simulink model "lab4_E1"  (R2020a)
settings: Solver=FixedStepAuto  StartTime=0.0  StopTime=100  FixedStep=0.001  RelTol=1e-3
values from neighbouring files (symbols this model uses):
  y_r = 1    [lab8.mat]
undefined symbols (not defined in the file or in its folder): h, K, M, x_1_0, x_2_0, x_3_0
settings Model: Creator=bruno  LastModifiedBy=bruno

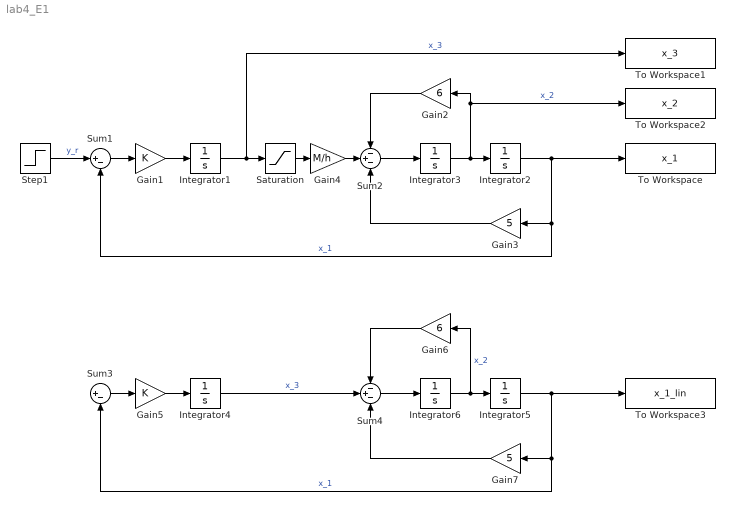
== system lab4_E1 ==
  Gain1 : Gain  Gain=K
  Gain2 : Gain  Gain=6
  Gain3 : Gain  Gain=5
  Gain4 : Gain  Gain=M/h
  Gain5 : Gain  Gain=K
  Gain6 : Gain  Gain=6
  Gain7 : Gain  Gain=5
  Integrator1 : Integrator  InitialCondition=x_3_0
  Integrator2 : Integrator  InitialCondition=x_1_0
  Integrator3 : Integrator  InitialCondition=x_2_0
  Integrator4 : Integrator  InitialCondition=x_3_0
  Integrator5 : Integrator  InitialCondition=x_1_0
  Integrator6 : Integrator  InitialCondition=x_2_0
  Saturation : Saturate  UpperLimit=h  LowerLimit=-h
  Step1 : Step  Time=0  After=y_r  SampleTime=0
  Sum1 : Sum  Inputs=|+-
  Sum2 : Sum  Inputs=-+-
  Sum3 : Sum  Inputs=|+-
  Sum4 : Sum  Inputs=-+-
  To Workspace : ToWorkspace  VariableName=x_1  SaveFormat=Timeseries  SampleTime=-1
  To Workspace1 : ToWorkspace  VariableName=x_3  SaveFormat=Timeseries  SampleTime=-1
  To Workspace2 : ToWorkspace  VariableName=x_2  SaveFormat=Timeseries  SampleTime=-1
  To Workspace3 : ToWorkspace  VariableName=x_1_lin  SaveFormat=Timeseries  SampleTime=-1
  wires:
  Gain1/1 -> Integrator1/1
  Sum1/1 -> Gain1/1
  Integrator3/1 -> To Workspace2/1, Gain2/1, Integrator2/1  "x_2"
  Sum2/1 -> Integrator3/1
  Gain2/1 -> Sum2/1
  Gain3/1 -> Sum2/3
  Integrator2/1 -> To Workspace/1, Gain3/1, Sum1/2  "x_1"
  Integrator1/1 -> To Workspace1/1, Saturation/1  "x_3"
  Saturation/1 -> Gain4/1
  Gain4/1 -> Sum2/2
  Integrator4/1 -> Sum4/2  "x_3"
  Integrator5/1 -> To Workspace3/1, Sum3/2, Gain7/1  "x_1"
  Gain7/1 -> Sum4/3
  Gain6/1 -> Sum4/1
  Sum4/1 -> Integrator6/1
  Integrator6/1 -> Integrator5/1, Gain6/1  "x_2"
  Step1/1 -> Sum1/1  "y_r"
  Sum3/1 -> Gain5/1
  Gain5/1 -> Integrator4/1
